simulink model "PreliminarySim"  (R2021a)
settings: Solver=VariableStepAuto  StartTime=0.0  StopTime=10.0  RelTol=1e-3
libraries: ee_lib x10, fl_lib x7, nesl_utility x2
settings Model: Creator=caryp  LastModifiedBy=caryp

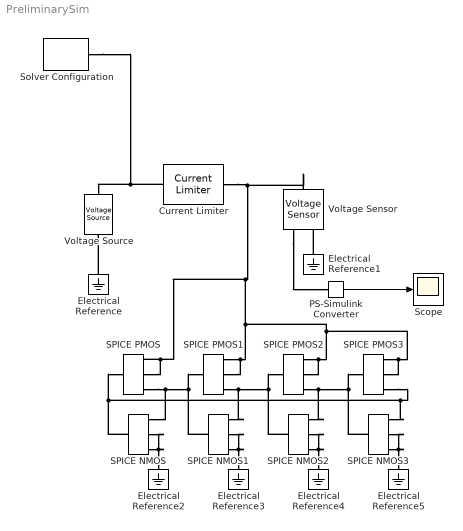
== system PreliminarySim ==
  Current Limiter : ee_lib/Semiconductors & Converters/Current Limiter  iLim=30 mA  vLim=0.1 V  gLim=1e-3 1/Ohm  thermal_mass=100 J/K  initial_temperature=298.15 K
      settings: SourceProductBaseCode=PS  InternalSimscapePortConfiguration="{\"Bottom\":[],\"Left\":[{\"id\":\"p\",\"label\":\"+\",\"type\":\"foundation.electrical.electrical\"}],\"Right\":[{\"id\":\"n\",\"label\":\"-\",\"type\":\"foundation.electrical.electrical\"}],\"Top\":[]}"
  Electrical Reference{,1..5} (6 alike) : fl_lib/Electrical/Electrical Elements/Electrical Reference
  PS-Simulink Converter : nesl_utility/PS-Simulink Converter  PhysicalDomain=network_engine_domain  SubClassName=ps_output  LeftPortType=input  RightPortType=output  PseudoPeriodic=off  Frequencies=[]  Unit=inherit  AffineConversion=off
      settings: SourceProductBaseCode=PW,SS
  SPICE NMOS{,1..3} (4 alike) : ee_lib/Additional Components/SPICE Semiconductors/SPICE NMOS  AREA=1.0  SCALE=1  LENGTH=1e-4 m  WIDTH=1e-4 m  AD=0 m^2  AS=0 m^2  PD=0 m  PS=0 m  NRD=0  NRS=0  LEVEL=1  VTO=2.5 V  KP=2e-5 A/V^2  GAMMA=0 V^0.50000  PHI=0.6 V  LAMBDA=0 1/V  RD=0 Ohm  RS=0 Ohm  Ci_param=ee.enum.intrinsicCapacitance.none  Cov_param=ee.enum.includeCapacitance.no  CGSO=0 F/m  CGDO=0 F/m  CGBO=0 F/m  C_param=ee.enum.includeCapacitance.no  CBD=0 F  CBS=0 F  IS=1 A  N=1  PB=0.8 V  RSH=0 Ohm  CJ=0 F/m^2  MJ=0.5  CJSW=0 F/m  MJSW=0.5  JS=0 A/m^2  TOX=1e-7 m  LD=0 m  U0=600 cm^2/s/V  FC=0.5  NSUB=NaN 1/cm^3  TPG=1  NSS=NaN 1/cm^2  DELTA=0  VMAX=0 m/s  XJ=0 m  NFS=0 1/cm^2  ETA=0  THETA=0 1/V  KAPPA=0.2  T_param=1  TFIXED=300.15 K  TMEAS=300.15 K  TOFFSET=0 K  UEXP=0  UCRIT=1e4 V/cm  NEFF=1  IC_given=ee.enum.initialCondition.no  ICVDS=0 V  ICVGS=0 V  ICVBS=0 V  MTYPE=1
      settings: SourceProductBaseCode=PS  InternalSimscapePortConfiguration="{\"Bottom\":[],\"Left\":[{\"id\":\"gx\",\"label\":\"\",\"type\":\"foundation.electrical.electrical\"}],\"Right\":[{\"id\":\"dx\",\"label\":\"\",\"type\":\"foundation.electrical.electrical\"},{\"id\":\"bx\",\"label\":\"\",\"type\":\"foundation.electrical.electrical\"},{\"id\":\"sx\",\"label\":\"\",\"type\":\"foundation.electrical.electrical\"}],\"Top\":[]}"
  SPICE PMOS : ee_lib/Additional Components/SPICE Semiconductors/SPICE PMOS  AREA=1.0  SCALE=1  LENGTH=1e-4 m  WIDTH=1e-4 m  AD=0 m^2  AS=0 m^2  PD=0 m  PS=0 m  NRD=0  NRS=0  LEVEL=3  VTO=2.5 V  KP=2e-5 A/V^2  GAMMA=0 V^0.50000  PHI=0.6 V  LAMBDA=0 1/V  RD=0 Ohm  RS=0 Ohm  Ci_param=ee.enum.intrinsicCapacitance.none  Cov_param=ee.enum.includeCapacitance.no  CGSO=0 F/m  CGDO=0 F/m  CGBO=0 F/m  C_param=ee.enum.includeCapacitance.no  CBD=0 F  CBS=0 F  IS=1 A  N=1  PB=0.8 V  RSH=0 Ohm  CJ=0 F/m^2  MJ=0.5  CJSW=0 F/m  MJSW=0.5  JS=0 A/m^2  TOX=1e-7 m  LD=0 m  U0=600 cm^2/s/V  FC=0.5  NSUB=NaN 1/cm^3  TPG=1  NSS=NaN 1/cm^2  DELTA=0  VMAX=0 m/s  XJ=0 m  NFS=0 1/cm^2  ETA=0  THETA=0 1/V  KAPPA=0.2  T_param=1  TFIXED=300.15 K  TMEAS=300.15 K  TOFFSET=0 K  UEXP=0  UCRIT=1e4 V/cm  NEFF=1  IC_given=ee.enum.initialCondition.no  ICVDS=0 V  ICVGS=0 V  ICVBS=0 V  MTYPE=-1
      settings: SourceProductBaseCode=PS  InternalSimscapePortConfiguration="{\"Bottom\":[],\"Left\":[{\"id\":\"gx\",\"label\":\"\",\"type\":\"foundation.electrical.electrical\"}],\"Right\":[{\"id\":\"dx\",\"label\":\"\",\"type\":\"foundation.electrical.electrical\"},{\"id\":\"bx\",\"label\":\"\",\"type\":\"foundation.electrical.electrical\"},{\"id\":\"sx\",\"label\":\"\",\"type\":\"foundation.electrical.electrical\"}],\"Top\":[]}"
  SPICE PMOS1 : ee_lib/Additional Components/SPICE Semiconductors/SPICE PMOS  AREA=1.0  SCALE=1  LENGTH=1e-4 m  WIDTH=1e-4 m  AD=0 m^2  AS=0 m^2  PD=0 m  PS=0 m  NRD=0  NRS=0  LEVEL=1  VTO=2.5 V  KP=2e-5 A/V^2  GAMMA=0 V^0.50000  PHI=0.6 V  LAMBDA=0 1/V  RD=0 Ohm  RS=0 Ohm  Ci_param=ee.enum.intrinsicCapacitance.none  Cov_param=ee.enum.includeCapacitance.no  CGSO=0 F/m  CGDO=0 F/m  CGBO=0 F/m  C_param=ee.enum.includeCapacitance.no  CBD=0 F  CBS=0 F  IS=1 A  N=1  PB=0.8 V  RSH=0 Ohm  CJ=0 F/m^2  MJ=0.5  CJSW=0 F/m  MJSW=0.5  JS=0 A/m^2  TOX=1e-7 m  LD=0 m  U0=600 cm^2/s/V  FC=0.5  NSUB=NaN 1/cm^3  TPG=1  NSS=NaN 1/cm^2  DELTA=0  VMAX=0 m/s  XJ=0 m  NFS=0 1/cm^2  ETA=0  THETA=0 1/V  KAPPA=0.2  T_param=1  TFIXED=300.15 K  TMEAS=300.15 K  TOFFSET=0 K  UEXP=0  UCRIT=1e4 V/cm  NEFF=1  IC_given=ee.enum.initialCondition.no  ICVDS=0 V  ICVGS=0 V  ICVBS=0 V  MTYPE=-1
      settings: SourceProductBaseCode=PS  InternalSimscapePortConfiguration="{\"Bottom\":[],\"Left\":[{\"id\":\"gx\",\"label\":\"\",\"type\":\"foundation.electrical.electrical\"}],\"Right\":[{\"id\":\"dx\",\"label\":\"\",\"type\":\"foundation.electrical.electrical\"},{\"id\":\"bx\",\"label\":\"\",\"type\":\"foundation.electrical.electrical\"},{\"id\":\"sx\",\"label\":\"\",\"type\":\"foundation.electrical.electrical\"}],\"Top\":[]}"
  SPICE PMOS2 : ee_lib/Additional Components/SPICE Semiconductors/SPICE PMOS  AREA=1.0  SCALE=1  LENGTH=1e-4 m  WIDTH=1e-4 m  AD=0 m^2  AS=0 m^2  PD=0 m  PS=0 m  NRD=0  NRS=0  LEVEL=1  VTO=2.5 V  KP=2e-5 A/V^2  GAMMA=0 V^0.50000  PHI=0.6 V  LAMBDA=0 1/V  RD=0 Ohm  RS=0 Ohm  Ci_param=ee.enum.intrinsicCapacitance.none  Cov_param=ee.enum.includeCapacitance.no  CGSO=0 F/m  CGDO=0 F/m  CGBO=0 F/m  C_param=ee.enum.includeCapacitance.no  CBD=0 F  CBS=0 F  IS=1 A  N=1  PB=0.8 V  RSH=0 Ohm  CJ=0 F/m^2  MJ=0.5  CJSW=0 F/m  MJSW=0.5  JS=0 A/m^2  TOX=1e-7 m  LD=0 m  U0=600 cm^2/s/V  FC=0.5  NSUB=NaN 1/cm^3  TPG=1  NSS=NaN 1/cm^2  DELTA=0  VMAX=0 m/s  XJ=0 m  NFS=0 1/cm^2  ETA=0  THETA=0 1/V  KAPPA=0.2  T_param=1  TFIXED=300.15 K  TMEAS=300.15 K  TOFFSET=0 K  UEXP=0  UCRIT=1e4 V/cm  NEFF=1  IC_given=ee.enum.initialCondition.no  ICVDS=0 V  ICVGS=0 V  ICVBS=0 V  MTYPE=-1
      settings: SourceProductBaseCode=PS  InternalSimscapePortConfiguration="{\"Bottom\":[],\"Left\":[{\"id\":\"gx\",\"label\":\"\",\"type\":\"foundation.electrical.electrical\"}],\"Right\":[{\"id\":\"dx\",\"label\":\"\",\"type\":\"foundation.electrical.electrical\"},{\"id\":\"bx\",\"label\":\"\",\"type\":\"foundation.electrical.electrical\"},{\"id\":\"sx\",\"label\":\"\",\"type\":\"foundation.electrical.electrical\"}],\"Top\":[]}"
  SPICE PMOS3 : ee_lib/Additional Components/SPICE Semiconductors/SPICE PMOS  AREA=1.0  SCALE=1  LENGTH=1e-4 m  WIDTH=1e-4 m  AD=0 m^2  AS=0 m^2  PD=0 m  PS=0 m  NRD=0  NRS=0  LEVEL=1  VTO=2.5 V  KP=2e-5 A/V^2  GAMMA=0 V^0.50000  PHI=0.6 V  LAMBDA=0 1/V  RD=0 Ohm  RS=0 Ohm  Ci_param=ee.enum.intrinsicCapacitance.none  Cov_param=ee.enum.includeCapacitance.no  CGSO=0 F/m  CGDO=0 F/m  CGBO=0 F/m  C_param=ee.enum.includeCapacitance.no  CBD=0 F  CBS=0 F  IS=1 A  N=1  PB=0.8 V  RSH=0 Ohm  CJ=0 F/m^2  MJ=0.5  CJSW=0 F/m  MJSW=0.5  JS=0 A/m^2  TOX=1e-7 m  LD=0 m  U0=600 cm^2/s/V  FC=0.5  NSUB=NaN 1/cm^3  TPG=1  NSS=NaN 1/cm^2  DELTA=0  VMAX=0 m/s  XJ=0 m  NFS=0 1/cm^2  ETA=0  THETA=0 1/V  KAPPA=0.2  T_param=1  TFIXED=300.15 K  TMEAS=300.15 K  TOFFSET=0 K  UEXP=0  UCRIT=1e4 V/cm  NEFF=1  IC_given=ee.enum.initialCondition.no  ICVDS=0 V  ICVGS=0 V  ICVBS=0 V  MTYPE=-1
      settings: SourceProductBaseCode=PS  InternalSimscapePortConfiguration="{\"Bottom\":[],\"Left\":[{\"id\":\"gx\",\"label\":\"\",\"type\":\"foundation.electrical.electrical\"}],\"Right\":[{\"id\":\"dx\",\"label\":\"\",\"type\":\"foundation.electrical.electrical\"},{\"id\":\"bx\",\"label\":\"\",\"type\":\"foundation.electrical.electrical\"},{\"id\":\"sx\",\"label\":\"\",\"type\":\"foundation.electrical.electrical\"}],\"Top\":[]}"
  Scope : Scope
  Solver Configuration : nesl_utility/Solver Configuration  PhysicalDomain=network_engine_domain  SubClassName=solver  LeftPortType=input  RightPortType=generic  Tones=[]  Harmonics=[]  SimulateNoise=off  Profile=off  UseLocalSampling=off  EnableSwitchedLinearOptims=on  FrequencyDomain=off  UseCCode=off  RelTol=0.001  AbsTol=1e-06  MinStep=1e-09  ToWorkspace=off  RevertToSquareIcSolve=off  NumHomotopyIterations=100  PhasorMode=off  PhasorModeNumHarmonics=1  DoDC=on  ResidualTolerance=1e-09  UseLocalSolver=off  LocalSolverChoice=NE_BACKWARD_EULER_ADVANCER  LocalSolverSampleTime=0.001  DoFixedCost=off  MaxNonlinIter=3  MaxModeIter=2  ComputeImpulses=off  ImpulseIterations=2  LinearAlgebra=Full  EquationFormulation=NE_TIME_EF  DelaysMemoryBudget=1024  AutomaticFiltering=on  FilteringTimeConstant=0.001  PartitionStorageMethod=AS_NEEDED  PartitionMemoryBudget=1024  PartitionMethod=ROBUST
      settings: SourceProductBaseCode=PW,SS
  Voltage Sensor : fl_lib/Electrical/Electrical Sensors/Voltage Sensor
  Voltage Source : ee_lib/Sources/Voltage Source  dc_voltage=5 V  ac_voltage=0 V  ac_shift=0 rad  ac_frequency=60 Hz  noise_mode=0  PSD=0 V^2/Hz  repeatability=1  auto_seed=3499211588  user_seed=0  sample_time=1e-3 s  i_specify=off  i_priority=None  i=0 A  i_nominal_specify=off  i_nominal_unit=A  i_nominal_value=1  v_specify=off  v_priority=None  v=0 V  v_nominal_specify=off  v_nominal_unit=V  v_nominal_value=1
  wires:
  PS-Simulink Converter/1 -> Scope/1
  connections:
  Current Limiter/LConn1 -- Solver Configuration/RConn1 -- Voltage Source/LConn1
  Voltage Sensor/RConn1 -- PS-Simulink Converter/LConn1
  Electrical Reference/LConn1 -- Voltage Source/RConn1
  Electrical Reference1/LConn1 -- Voltage Sensor/RConn2
  SPICE NMOS/RConn3 -- Electrical Reference2/LConn1 -- SPICE NMOS/RConn2
  SPICE NMOS/LConn1 -- SPICE PMOS3/RConn3 -- SPICE NMOS3/RConn1 -- SPICE PMOS/LConn1
  SPICE NMOS1/RConn3 -- Electrical Reference3/LConn1 -- SPICE NMOS1/RConn2
  SPICE NMOS1/LConn1 -- SPICE NMOS/RConn1 -- SPICE PMOS/RConn3 -- SPICE PMOS1/LConn1
  SPICE NMOS2/RConn3 -- Electrical Reference4/LConn1 -- SPICE NMOS2/RConn2
  SPICE NMOS2/LConn1 -- SPICE NMOS1/RConn1 -- SPICE PMOS1/RConn3 -- SPICE PMOS2/LConn1
  SPICE NMOS3/RConn3 -- Electrical Reference5/LConn1 -- SPICE NMOS3/RConn2
  SPICE NMOS3/LConn1 -- SPICE NMOS2/RConn1 -- SPICE PMOS2/RConn3 -- SPICE PMOS3/LConn1
  Current Limiter/RConn1 -- Voltage Sensor/LConn1 -- SPICE PMOS3/RConn2 -- SPICE PMOS3/RConn1 -- SPICE PMOS2/RConn2 -- SPICE PMOS2/RConn1 -- SPICE PMOS1/RConn2 -- SPICE PMOS1/RConn1 -- SPICE PMOS/RConn2 -- SPICE PMOS/RConn1
